simulink subsystem "Normal_Forces_and_Moments"  (R2024b)
settings: Solver=VariableStepAuto  StartTime=0.0  StopTime=10.0  RelTol=1e-3
values from neighbouring files (symbols this model uses):
  Af = (Cr + Ct) * span / 2    [Barrowman_Equations.m]    (also in barrowaman.mat = 0.042987)
  CnalfaBody = 2.2 * lTubo    [Barrowman_Equations.m]    (also in barrowaman.mat = 7.5064)
  CnAlfaNose = 2 * pi * (r0^2) / Ar    [Barrowman_Equations.m]    (also in barrowaman.mat = 2)
  Cnalfat = Cnalfat * (1 + r0/(span + r0))    [Barrowman_Equations.m]    (also in barrowaman.mat = 12.382152073)
  Cnalfat_canard = Cnalfat_canard * (1 + r0/(span_canard + r0))    [Barrowman_Equations.m]    (also in barrowaman.mat = 2.80482456232)
  CnAlfaTail = 0    [Barrowman_Equations.m]    (also in barrowaman.mat = -0.303324099723)
  h = 0.0794    [barrowaman.mat]
  logiva = 0.638    [barrowaman.mat]
  Lr = 0.152    [barrowaman.mat]
  lTubo = 3.412    [barrowaman.mat]
  N = 3    [barrowaman.mat]
  pos_aletas = -3.7003    [barrowaman.mat]
  XB = -(logiva - logiva/2)    [Barrowman_Equations.m]    (also in barrowaman.mat = -0.319)
  Xtail = 0    [Barrowman_Equations.m]    (also in barrowaman.mat = -4.00975616438)
  XTB = pos_aletas - (sweep / 3) * ( (Cr + 2 * Ct) / (Cr + Ct) ) + (1/6) * (Cr + Ct - Cr * Ct / (Cr + Ct))    [Barrowman_Equations.m]    (also in barrowaman.mat = -3.65215541753)
  XTB_canard = x_cg    [Barrowman_Equations.m]    (also in barrowaman.mat = -3.17)
settings Model: Creator=joedo  LastModifiedBy=joedo

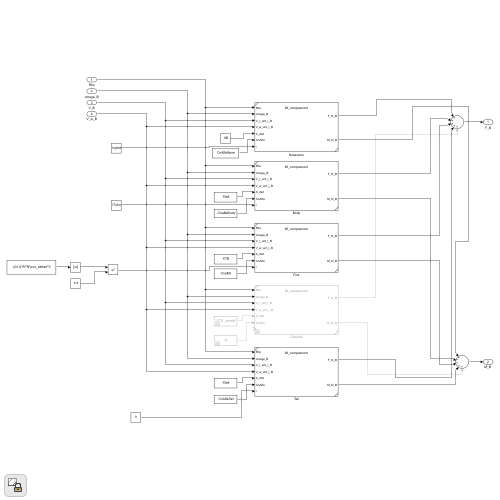
[thumbnail: Simulink's stored preview of the top-level diagram]
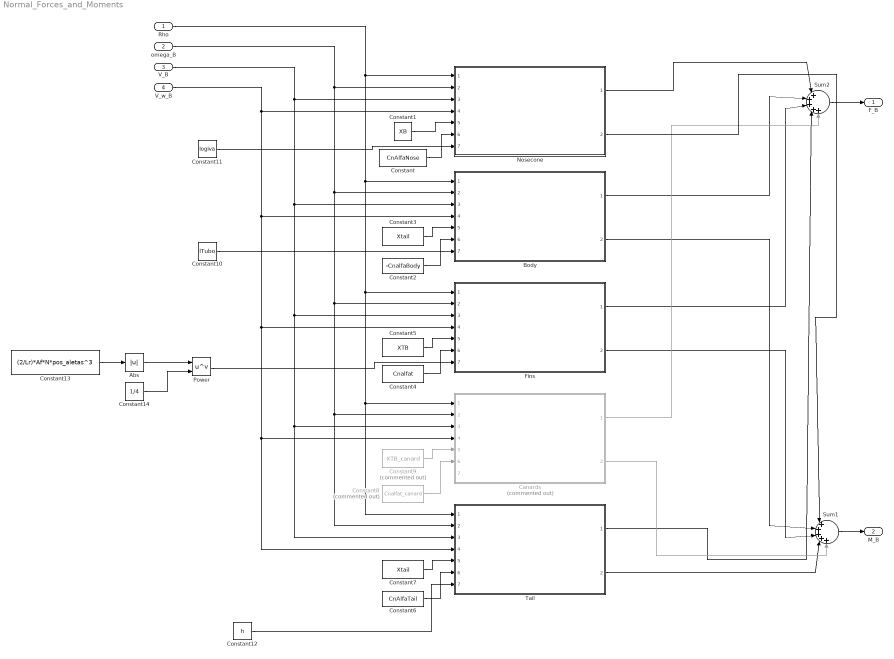
== system Normal_Forces_and_Moments ==
  Rho : Inport
  omega_B : Inport  Port=2
  "V_B " : Inport  Port=3
  V_w_B : Inport  Port=4
  Abs : Abs  SaturateOnIntegerOverflow=off
  Body : Subsystem  ReferencedSubsystem=lift_compoenent
  Canards : Subsystem  Commented=on  ReferencedSubsystem=lift_compoenent
  Constant : Constant  Value=CnAlfaNose
  Constant1 : Constant  Value=XB
  Constant10 : Constant  Value=lTubo
  Constant11 : Constant  Value=logiva
  Constant12 : Constant  Value=h
  Constant13 : Constant  Value=(2/Lr)*Af*N*pos_aletas^3
  Constant14 : Constant  Value=1/4
  Constant2 : Constant  Value=-CnalfaBody
  Constant3 : Constant  Value=Xtail
  Constant4 : Constant  Value=Cnalfat
  Constant5 : Constant  Value=XTB
  Constant6 : Constant  Value=CnAlfaTail
  Constant7 : Constant  Value=Xtail
  Constant8 : Constant  Commented=on  Value=Cnalfat_canard
  Constant9 : Constant  Commented=on  Value=XTB_canard
  Fins : Subsystem  ReferencedSubsystem=lift_compoenent
  Nosecone : Subsystem  ReferencedSubsystem=lift_compoenent
  Power : Math  Operator=pow
  Sum1 : Sum  Inputs=|+++++
  Sum2 : Sum  Inputs=|+++++
  Tail : Subsystem  ReferencedSubsystem=lift_compoenent
  "F_B " : Outport  VectorParamsAs1DForOutWhenUnconnected=off
  "M_B " : Outport  Port=2  VectorParamsAs1DForOutWhenUnconnected=off
  wires:
  "V_B "/1 -> Nosecone/3, Body/3, Fins/3, Canards/3, Tail/3
  omega_B/1 -> Nosecone/2, Body/2, Fins/2, Canards/2, Tail/2
  V_w_B/1 -> Nosecone/4, Body/4, Fins/4, Canards/4, Tail/4
  Rho/1 -> Fins/1, Canards/1, Tail/1, Body/1, Nosecone/1
  Sum1/1 -> "M_B "/1
  Sum2/1 -> "F_B "/1
  Body/1 -> Sum2/2
  Body/2 -> Sum1/2
  Fins/1 -> Sum2/3
  Fins/2 -> Sum1/3
  Tail/1 -> Sum2/4
  Tail/2 -> Sum1/4
  Canards/1 -> Sum2/5
  Canards/2 -> Sum1/5
  Constant/1 -> Nosecone/6
  Constant1/1 -> Nosecone/5
  Nosecone/1 -> Sum2/1
  Nosecone/2 -> Sum1/1
  Constant2/1 -> Body/6
  Constant3/1 -> Body/5
  Constant5/1 -> Fins/5
  Constant4/1 -> Fins/6
  Constant7/1 -> Tail/5
  Constant6/1 -> Tail/6
  Constant9/1 -> Canards/5
  Constant8/1 -> Canards/6
  Constant11/1 -> Nosecone/7
  Constant10/1 -> Body/7
  Constant12/1 -> Tail/7
  Constant13/1 -> Abs/1
  Abs/1 -> Power/1
  Constant14/1 -> Power/2
  Power/1 -> Fins/7
